simulink model "motor"  (R2016b)
settings: Solver=VariableStepAuto  StartTime=0.0  StopTime=0.10  RelTol=1e-3
settings Model: Creator=Biscuit  LastModifiedBy=Biscuit

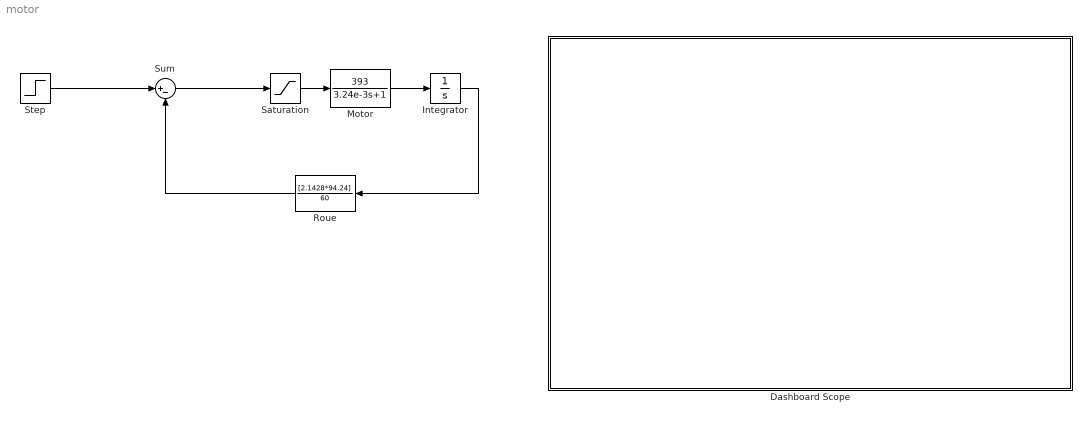
== system motor ==
  Dashboard Scope : Subsystem  DialogController=hmiCreateDDGDialog  IsWebBlock=on  mask(MWDashboardBlock){webBlockId=47472bb8-729e-4d6f-be7f-833571e2985a, webBlockType=sdiscope, ShowInitialText=on, HMISrcModelName=untitled}
      mask prompts: webBlockId "WebBlock Id"; webBlockType "WebBlock Type"; HMISrcModelName "Source Model"
      mask help: SimulinkHMI:dialogs:HMIScopeDialogDesc
      mask Help: helpview([docroot '/mapfiles/simulink.map'], 'hmi_scope')
      mask Display:
      | if strcmp(get_param(bdroot(gcb),'BlockDiagramType'), 'library')
      |     image([(matlabroot) '/toolbox/simulink/hmi/icons/DashboardScope.png']);
      | end
  Integrator : Integrator
  Motor : TransferFcn  Numerator=[393]  Denominator=[3.24e-3 1]
  Roue : TransferFcn  Numerator=[2.1428*94.24]  Denominator=[60]
  Saturation : Saturate  UpperLimit=18  LowerLimit=0
  Step : Step  Time=0  After=100  SampleTime=0
  Sum : Sum  Inputs=|+-
  wires:
  Saturation/1 -> Motor/1
  Motor/1 -> Integrator/1
  Sum/1 -> Saturation/1
  Integrator/1 -> Roue/1
  Roue/1 -> Sum/2
  Step/1 -> Sum/1

== system motor/Dashboard Scope ==
